simulink model "Linearisierung3_RoboKomplettmodellUebersicht_Sim"  (R2017a)
settings: Solver=VariableStepAuto  StartTime=0.0  StopTime=10.0  RelTol=1e-3
values from neighbouring files (symbols this model uses):
  c = 1    [Linearisierung3_Robo.m]
  g = 9.81    [Linearisierung3_Robo.m]
  K = 300    [Linearisierung3_Robo.m]
  l = 1    [Linearisierung3_Robo.m]
  m = 7    [Linearisierung3_Robo.m]
  T = 0.1    [Linearisierung3_Robo.m]
settings Model: Creator=jonas  LastModifiedBy=jonas

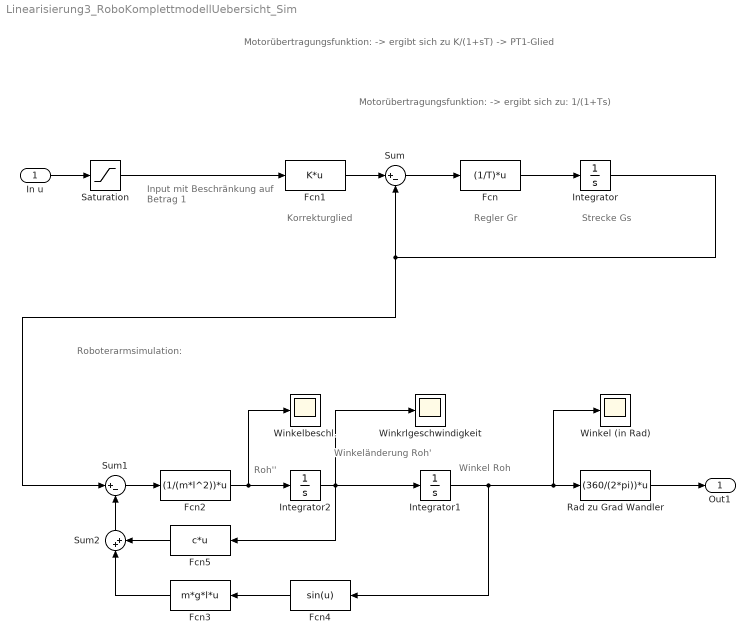
== system Linearisierung3_RoboKomplettmodellUebersicht_Sim ==
  note: Roboterarmsimulation:
  note: Strecke Gs
  note: Input
      | mit Beschränkung
      | auf Betrag 1
  note: Korrekturglied
  note: Motorübertragungsfunktion:
      |  -> ergibt sich zu: 1/(1+Ts)
  note: Regler Gr
  note: Motorübertragungsfunktion:
      |  -> ergibt sich zu K/(1+sT)
      |  -> PT1-Glied
  note: Winkel Roh
  note: Winkeländerung
      | Roh'
  note: Roh''
  "In u " : Inport
  Fcn : Fcn  Expr=(1/T)*u
  Fcn1 : Fcn  Expr=K*u
  Fcn2 : Fcn  Expr=(1/(m*l^2))*u
  Fcn3 : Fcn  Expr=m*g*l*u
  Fcn4 : Fcn  Expr=sin(u)
  Fcn5 : Fcn  Expr=c*u
  Integrator : Integrator
  Integrator1 : Integrator
  Integrator2 : Integrator
  Rad zu Grad Wandler : Fcn  Expr=(360/(2*pi))*u
  Saturation : Saturate  UpperLimit=1  LowerLimit=-1
  Sum : Sum  Inputs=|+-
  Sum1 : Sum  Inputs=|+-
  Sum2 : Sum  Inputs=|++
  "Winkel (in Rad) " : Scope
  Winkelbeschl. : Scope
  "Winkrlgeschwindigkeit " : Scope
  Out1 : Outport
  wires:
  Fcn/1 -> Integrator/1
  Saturation/1 -> Fcn1/1
  Integrator/1 -> Sum/2, Sum1/1
  Sum/1 -> Fcn/1
  Fcn1/1 -> Sum/1
  "In u "/1 -> Saturation/1
  Fcn4/1 -> Fcn3/1
  Sum2/1 -> Sum1/2
  Sum1/1 -> Fcn2/1
  Integrator1/1 -> "Winkel (in Rad) "/1, Rad zu Grad Wandler/1, Fcn4/1
  Rad zu Grad Wandler/1 -> Out1/1
  Fcn5/1 -> Sum2/2
  Fcn2/1 -> Integrator2/1, Winkelbeschl./1
  Fcn3/1 -> Sum2/1
  Integrator2/1 -> "Winkrlgeschwindigkeit "/1, Fcn5/1, Integrator1/1
